simulink model "framework_sim"  (R2019b)
settings: Solver=FixedStepDiscrete  StartTime=T0  StopTime=Tf  FixedStep=Ts  EnableMultiTasking=on
model workspace (MAT data in the model file):
  aKalman = Simulink.Parameter
  aKalman.DataType = 'auto'
  aKalman.Dimensions = [0 0]
  slipEnabler = Simulink.Parameter
  slipEnabler.DataType = 'auto'
  slipEnabler.Dimensions = [0 0]
values from neighbouring files (symbols this model uses):
  enable_onlinePlots = 0    [main_framework.m]
  enable_zoom = 0    [main_framework.m]
  HLP_sampleTime = planner.replan_time    [main_framework.m]
  Kb = 10    [main_framework.m]
  Kd_vals = PID_Gain_Scheduling(:,4)    [main_framework.m]
  Ki_vals = PID_Gain_Scheduling(:,3)    [main_framework.m]
  Kp_vals = PID_Gain_Scheduling(:,2)    [main_framework.m]
  latContr_select = 4    [select_lateralController.m]
  mapObjects = scenario.scenario_data.mapObjects    [main_framework.m]
  N_vals = PID_Gain_Scheduling(:,5)    [main_framework.m]
  refRoute_fewPoints = referencePath_fewPoints.refRoute_fewPoints    [main_framework.m]    (also in refPath_poses_fewPoints.mat = [5 34.9682620653 63.3276365473 92.153562059 121.414282249 15; routePlanner.m = [x_cloth_refPath_fewPoints',y_cloth_refPath_fewPoints',theta)
  speed_vals_PID_sched = PID_Gain_Scheduling(:,1)    [main_framework.m]
  tau_D = vehicle_data.steering_system.tau_D    [dataAnalysis.m]    (also in main_framework.m)
  Ts = simulationPars.times.step_size    [main_framework.m]
  vehicle_data = getVehicleDataStruct()    [aeroModel.m]    (also in loadInitialConditions.m; longitSlipModel.m; main_framework.m; perfectAcker.m)
  X0 = loadInitialConditions    [main_framework.m]
undefined symbols (not defined in the file or in its folder): DiscIntNeverNeededParam, loadInitialPose
libraries: simulink_extras x16, drivingvehiclecontroller x2, simulink x1
(part 1 of 3)
settings Model: Creator=Edoardo  LastModifiedBy=Alvaro
settings DataIOCC: SaveFormat=Array  ReturnWorkspaceOutputs=off
settings OptimizationCC: DefaultParameterBehavior=Inlined  PassReuseOutputArgsAs=Individual arguments  MaxStackSize=64  EfficientTunableParamExpr=on
settings DebuggingCC: ReadBeforeWriteMsg=DisableAll  WriteAfterWriteMsg=DisableAll  WriteAfterReadMsg=DisableAll  MultiTaskDSMMsg=none  ParameterTunabilityLossMsg=error  PregeneratedLibrarySubsystemCodeDiagnostic=none  SFUnexpectedBacktrackingDiag=warning  SFNoUnconditionalDefaultTransitionDiag=warning  SFExecutionAtInitializationDiag=none  ArithmeticOperatorsInVariantConditions=warning
settings HardwareCC: ProdBitPerInt=16  ProdBitPerPointer=16  ProdBitPerSizeT=16  ProdBitPerPtrDiffT=16  ProdLargestAtomicFloat=None  ProdWordSize=16  ProdHWDeviceType=STMicroelectronics->ST10/Super10
settings ModelReferenceCC: UpdateModelReferenceTargets=IfOutOfDate  PropagateSignalLabelsOutOfModel=off
settings SFSimCC: SFSimEcho=off  SimUseLocalCustomCode=off  MATLABDynamicMemAlloc=off  CustomCodeUndefinedFunction=UseInterfaceOnly
settings RTWCC: SystemTargetFile=ert.tlc  TemplateMakefile=ert_default_tmf  GenerateReport=on  RetainRTWFile=on  RTWUseLocalCustomCode=off  Toolchain=GNU Tools for ARM Embedded Processors  BuildConfiguration=Faster Runs  IncludeHyperlinkInReport=on  LaunchReport=on  GenerateTraceInfo=on  GenerateTraceReport=on  GenerateTraceReportSl=on  GenerateTraceReportSf=on  GenerateTraceReportEml=on
settings CodeAppCC: ForceParamTrailComments=on  IgnoreCustomStorageClasses=off  OperatorAnnotations=on  SimulinkDataObjDesc=on  SFDataObjDesc=on  InsertBlockDesc=on
settings ERTTargetCC: CodeReplacementLibrary=ARM Cortex-M (Optimized)  SupportVariableSizeSignals=on  RootIOFormat=Structure reference  ERTCustomFileTemplate=example_file_process.tlc
settings ConfigComp: CovMetricSettings=dw  CovHtmlReporting=on  CovSaveCumulativeToWorkspaceVar=on  CovSaveSingleToWorkspaceVar=on  CovExternalEMLEnable=off

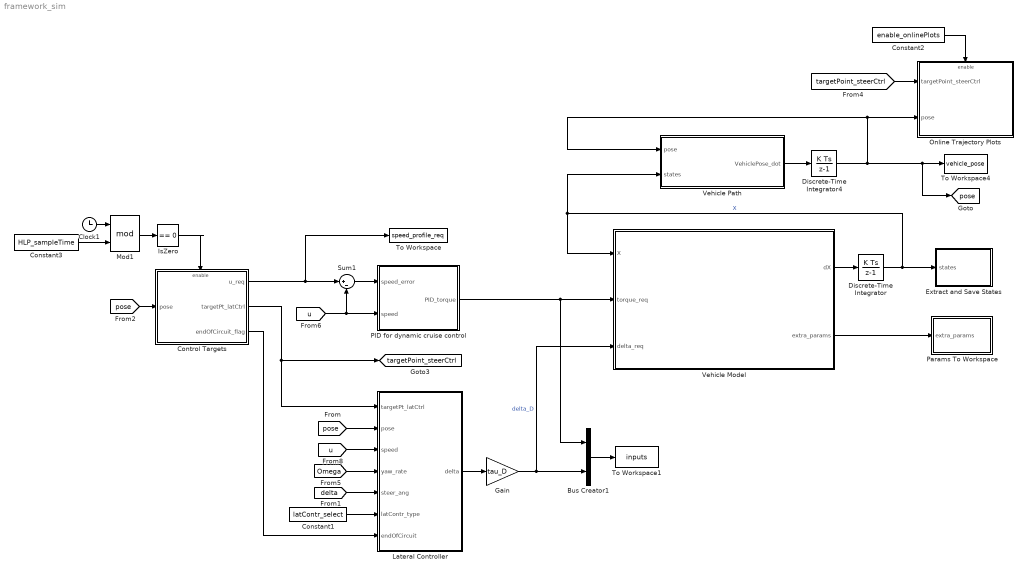
== system framework_sim ==
  Bus Creator1 : BusCreator  Inputs=2
  Clock1 : Clock
  Constant1 : Constant  Value=latContr_select
  Constant2 : Constant  Value=enable_onlinePlots
  Constant3 : Constant  Value=HLP_sampleTime
  Control Targets : Subsystem
  Discrete-Time Integrator : DiscreteIntegrator  gainval=1  InitialCondition=X0  SampleTime=-1  ICPrevOutput=DiscIntNeverNeededParam  ICPrevScaledInput=DiscIntNeverNeededParam
  Discrete-Time Integrator4 : DiscreteIntegrator  gainval=1  InitialCondition=loadInitialPose  SampleTime=-1  ICPrevOutput=DiscIntNeverNeededParam  ICPrevScaledInput=DiscIntNeverNeededParam
  Extract and Save States : Subsystem
  Gain : Gain  Gain=tau_D
  IsZero : simulink/Logic and Bit Operations/Compare To Zero  relop===  OutDataTypeStr=boolean
  Lateral Controller : Subsystem
  Mod1 : Math  Operator=mod  SaturateOnIntegerOverflow=on
  Online Trajectory Plots : Subsystem
      mask Display: image('/Users/mattiapiccinini/Documents/Google_Drive/PhD/Didattica/VDPC_EIT_2019_2020/Homework/Matlab_Maple/Homework_Autonomous_Drive_EIT/Scenario/example_path.png'); % Use "Edit Image" on toolstrip to change.
  PID for dynamic cruise control : Subsystem
  Params To Workspace : Subsystem
  Sum1 : Sum  Inputs=|+-
  To Workspace : ToWorkspace  VariableName=speed_profile_req  SaveFormat=Timeseries  SampleTime=-1
      settings: Save2DSignal=2-D array (concatenate along first dimension)
  To Workspace1 : ToWorkspace  VariableName=inputs  SaveFormat=Timeseries  SampleTime=-1
  To Workspace4 : ToWorkspace  VariableName=vehicle_pose  SampleTime=-1
      settings: Save2DSignal=2-D array (concatenate along first dimension)
  Vehicle Model : MATLAB Function  TreatAsAtomicUnit=on
  Vehicle Path : MATLAB Function  TreatAsAtomicUnit=on
  tag scope: pose=global, targetPoint_steerCtrl=global
  wires:
  [u] -> Sum1/2, PID for dynamic cruise control/2(speed)
  Vehicle Model/2(extra_params) -> Params To Workspace/1(extra_params)
  Discrete-Time Integrator/1 -> Extract and Save States/1(states), Vehicle Model/1(X), Vehicle Path/2(states)  "X"
  Vehicle Path/1(VehiclePose_dot) -> Discrete-Time Integrator4/1
  Discrete-Time Integrator4/1 -> [pose], To Workspace4/1, Online Trajectory Plots/2(pose), Vehicle Path/1(pose)
  Vehicle Model/1(dX) -> Discrete-Time Integrator/1
  Bus Creator1/1 -> To Workspace1/1
  PID for dynamic cruise control/1(PID_torque) -> Bus Creator1/1, Vehicle Model/2(torque_req)
  Sum1/1 -> PID for dynamic cruise control/1(speed_error)
  [targetPoint_steerCtrl] -> Online Trajectory Plots/1(targetPoint_steerCtrl)
  Gain/1 -> Vehicle Model/3(delta_req), Bus Creator1/2  "delta_D"
  Constant2/1 -> Online Trajectory Plots/Enable
  [pose] -> Lateral Controller/2(pose)
  [u] -> Lateral Controller/3(speed)
  Lateral Controller/1(delta) -> Gain/1
  Constant1/1 -> Lateral Controller/6(latContr_type)
  [Omega] -> Lateral Controller/4(yaw_rate)
  [delta] -> Lateral Controller/5(steer_ang)
  Control Targets/2(targetPt_latCtrl) -> Lateral Controller/1(targetPt_latCtrl), [targetPoint_steerCtrl]
  Control Targets/1(u_req) -> To Workspace/1, Sum1/1
  [pose] -> Control Targets/1(pose)
  Clock1/1 -> Mod1/1
  Constant3/1 -> Mod1/2
  Mod1/1 -> IsZero/1
  IsZero/1 -> Control Targets/Enable
  Control Targets/3(endOfCircuit_flag) -> Lateral Controller/7(endOfCircuit)

== system framework_sim/Control Targets ==
  pose : Inport
  Enable : EnablePort
  MATLAB System : MATLABSystem  System=setControlTargets  lateralController_type=latContr_select  purePursuit_lookAhead=purePursuitParams.lookAhead  clothoidBased_lookAhead=clothoidBasedParams.lookAhead  refRoute_points=refRoute_fewPoints  Lf=vehicle_data.vehicle.Lf  x_parkLot=mapObjects(1,1)  y_lowBound_parkLot=mapObjects(2,2)  y_uppBound_parkLot=mapObjects(1,2)  SimulateUsing=Interpreted execution
      mask Type: setControlTargets
      mask Display:
      | disp('setControlTargets');
      | port_label('input',1,'vehPose');
      | port_label('output',1,'targetPoint_latControl');
      | port_label('output',2,'speed_req');
      | port_label('output',3,'endOfCircuit');
  u_req : Outport  VectorParamsAs1DForOutWhenUnconnected=off
  targetPt_latCtrl : Outport  Port=2  VectorParamsAs1DForOutWhenUnconnected=off
  endOfCircuit_flag : Outport  Port=3  VectorParamsAs1DForOutWhenUnconnected=off
  wires:
  pose/1 -> MATLAB System/1
  MATLAB System/2 -> u_req/1
  MATLAB System/1 -> targetPt_latCtrl/1
  MATLAB System/3 -> endOfCircuit_flag/1

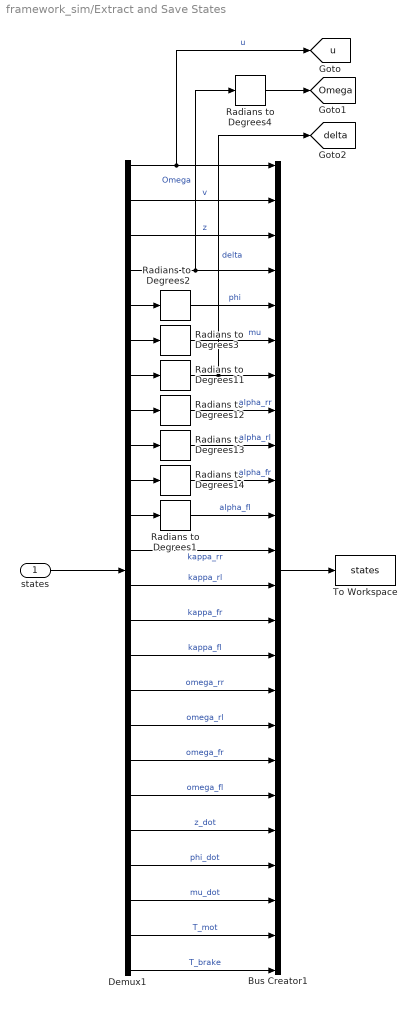
== system framework_sim/Extract and Save States ==
  states : Inport
  Bus Creator1 : BusCreator  Inputs=24
  Demux1 : Demux  Outputs=24
  Radians to Degrees{1..4,11..14} (8 alike) : simulink_extras/Transformations/Radians to Degrees
  To Workspace : ToWorkspace  VariableName=states  SaveFormat=Timeseries  SampleTime=-1
  tag scope: Omega=global, delta=global, u=global
  wires:
  Demux1/24 -> Bus Creator1/24  "T_brake"
  Demux1/13 -> Bus Creator1/13  "kappa_rl"
  Radians to Degrees12/1 -> Bus Creator1/8  "alpha_rr"
  Demux1/6 -> Radians to Degrees3/1
  Demux1/23 -> Bus Creator1/23  "T_mot"
  Demux1/19 -> Bus Creator1/19  "omega_fl"
  Demux1/8 -> Radians to Degrees12/1
  states/1 -> Demux1/1
  Demux1/14 -> Bus Creator1/14  "kappa_fr"
  Demux1/9 -> Radians to Degrees13/1
  Radians to Degrees11/1 -> Bus Creator1/7, [delta]  "delta"
  Demux1/15 -> Bus Creator1/15  "kappa_fl"
  Demux1/3 -> Bus Creator1/3  "z"
  Demux1/22 -> Bus Creator1/22  "mu_dot"
  Demux1/4 -> Bus Creator1/4, Radians to Degrees4/1  "Omega"
  Radians to Degrees3/1 -> Bus Creator1/6  "mu"
  Radians to Degrees1/1 -> Bus Creator1/11  "alpha_fl"
  Radians to Degrees2/1 -> Bus Creator1/5  "phi"
  Radians to Degrees13/1 -> Bus Creator1/9  "alpha_rl"
  Demux1/5 -> Radians to Degrees2/1
  Demux1/21 -> Bus Creator1/21  "phi_dot"
  Demux1/7 -> Radians to Degrees11/1
  Demux1/12 -> Bus Creator1/12  "kappa_rr"
  Demux1/17 -> Bus Creator1/17  "omega_rl"
  Demux1/2 -> Bus Creator1/2  "v"
  Demux1/20 -> Bus Creator1/20  "z_dot"
  Demux1/10 -> Radians to Degrees14/1
  Demux1/11 -> Radians to Degrees1/1
  Radians to Degrees14/1 -> Bus Creator1/10  "alpha_fr"
  Demux1/18 -> Bus Creator1/18  "omega_fr"
  Demux1/1 -> [u], Bus Creator1/1  "u"
  Demux1/16 -> Bus Creator1/16  "omega_rr"
  Bus Creator1/1 -> To Workspace/1
  Radians to Degrees4/1 -> [Omega]

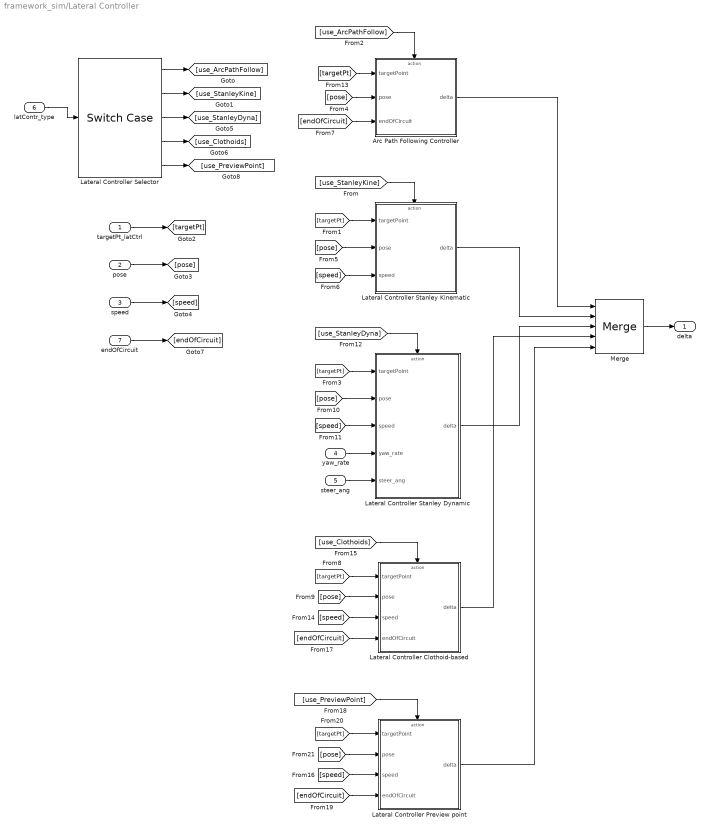
== system framework_sim/Lateral Controller ==
  targetPt_latCtrl : Inport
  pose : Inport  Port=2
  speed : Inport  Port=3
  yaw_rate : Inport  Port=4
  steer_ang : Inport  Port=5
  latContr_type : Inport  Port=6
  endOfCircuit : Inport  Port=7
  Arc Path Following Controller : Subsystem  TreatAsAtomicUnit=on
  Lateral Controller Clothoid-based : Subsystem  TreatAsAtomicUnit=on
  Lateral Controller Preview point : Subsystem  TreatAsAtomicUnit=on
  Lateral Controller Selector : SwitchCase  CaseConditions={1,2,3,4,5}  ShowDefaultCase=off
  Lateral Controller Stanley Dynamic : Subsystem  TreatAsAtomicUnit=on
  Lateral Controller Stanley Kinematic : Subsystem  TreatAsAtomicUnit=on
  Merge : Merge  Inputs=5
  delta : Outport  VectorParamsAs1DForOutWhenUnconnected=off
  wires:
  Arc Path Following Controller/1(delta) -> Merge/1
  latContr_type/1 -> Lateral Controller Selector/1
  Lateral Controller Stanley Kinematic/1(delta) -> Merge/2
  Merge/1 -> delta/1
  Lateral Controller Selector/1 -> [use_ArcPathFollow]
  [use_ArcPathFollow] -> Arc Path Following Controller/Action
  Lateral Controller Selector/2 -> [use_StanleyKine]
  [use_StanleyKine] -> Lateral Controller Stanley Kinematic/Action
  targetPt_latCtrl/1 -> [targetPt]
  [targetPt] -> Arc Path Following Controller/1(targetPoint)
  [targetPt] -> Lateral Controller Stanley Kinematic/1(targetPoint)
  pose/1 -> [pose]
  [pose] -> Arc Path Following Controller/2(pose)
  [pose] -> Lateral Controller Stanley Kinematic/2(pose)
  speed/1 -> [speed]
  [speed] -> Lateral Controller Stanley Kinematic/3(speed)
  Lateral Controller Selector/3 -> [use_StanleyDyna]
  [pose] -> Lateral Controller Stanley Dynamic/2(pose)
  [targetPt] -> Lateral Controller Stanley Dynamic/1(targetPoint)
  [speed] -> Lateral Controller Stanley Dynamic/3(speed)
  [use_StanleyDyna] -> Lateral Controller Stanley Dynamic/Action
  Lateral Controller Stanley Dynamic/1(delta) -> Merge/3
  yaw_rate/1 -> Lateral Controller Stanley Dynamic/4(yaw_rate)
  steer_ang/1 -> Lateral Controller Stanley Dynamic/5(steer_ang)
  [use_Clothoids] -> Lateral Controller Clothoid-based/Action
  [pose] -> Lateral Controller Clothoid-based/2(pose)
  [targetPt] -> Lateral Controller Clothoid-based/1(targetPoint)
  [speed] -> Lateral Controller Clothoid-based/3(speed)
  Lateral Controller Clothoid-based/1(delta) -> Merge/4
  Lateral Controller Selector/4 -> [use_Clothoids]
  [endOfCircuit] -> Arc Path Following Controller/3(endOfCircuit)
  [endOfCircuit] -> Lateral Controller Clothoid-based/4(endOfCircuit)
  endOfCircuit/1 -> [endOfCircuit]
  Lateral Controller Selector/5 -> [use_PreviewPoint]
  [pose] -> Lateral Controller Preview point/2(pose)
  [endOfCircuit] -> Lateral Controller Preview point/4(endOfCircuit)
  [use_PreviewPoint] -> Lateral Controller Preview point/Action
  [speed] -> Lateral Controller Preview point/3(speed)
  [targetPt] -> Lateral Controller Preview point/1(targetPoint)
  Lateral Controller Preview point/1(delta) -> Merge/5

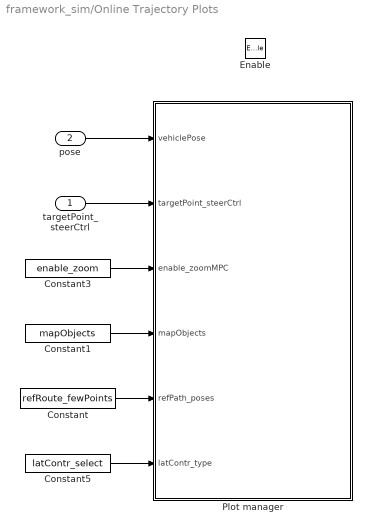
== system framework_sim/Online Trajectory Plots ==
  targetPoint_steerCtrl : Inport
  pose : Inport  Port=2
  Enable : EnablePort
  Constant : Constant  Value=refRoute_fewPoints
  Constant1 : Constant  Value=mapObjects
  Constant3 : Constant  Value=enable_zoom
  Constant5 : Constant  Value=latContr_select
  Plot manager : MATLAB Function  TreatAsAtomicUnit=on
  wires:
  targetPoint_steerCtrl/1 -> Plot manager/2(targetPoint_steerCtrl)
  Constant/1 -> Plot manager/5(refPath_poses)
  Constant3/1 -> Plot manager/3(enable_zoomMPC)
  pose/1 -> Plot manager/1(vehiclePose)
  Constant1/1 -> Plot manager/4(mapObjects)
  Constant5/1 -> Plot manager/6(latContr_type)

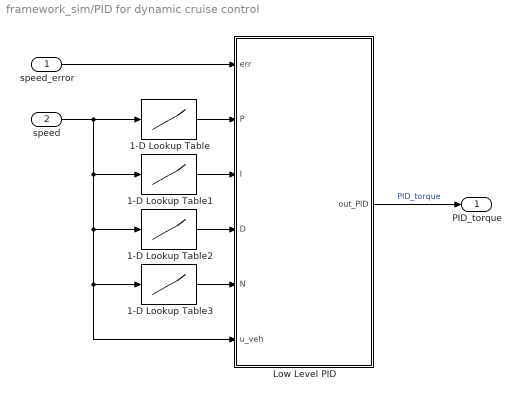
== system framework_sim/PID for dynamic cruise control ==
  speed_error : Inport
  speed : Inport  Port=2
  1-D Lookup Table : Lookup_n-D  NumberOfTableDimensions=1  BreakpointsForDimension1=speed_vals_PID_sched  BeginIndexSearchUsingPreviousIndexResult=on  Table=Kp_vals  ExtrapMethod=Clip  UseLastTableValue=on  InternalRulePriority=Speed  RndMeth=Simplest  InputSameDT=on
  1-D Lookup Table1 : Lookup_n-D  NumberOfTableDimensions=1  BreakpointsForDimension1=speed_vals_PID_sched  BeginIndexSearchUsingPreviousIndexResult=on  Table=Ki_vals  ExtrapMethod=Clip  UseLastTableValue=on  InternalRulePriority=Speed  RndMeth=Simplest  InputSameDT=on
  1-D Lookup Table2 : Lookup_n-D  NumberOfTableDimensions=1  BreakpointsForDimension1=speed_vals_PID_sched  BeginIndexSearchUsingPreviousIndexResult=on  Table=Kd_vals  ExtrapMethod=Clip  UseLastTableValue=on  InternalRulePriority=Speed  RndMeth=Simplest  InputSameDT=on
  1-D Lookup Table3 : Lookup_n-D  NumberOfTableDimensions=1  BreakpointsForDimension1=speed_vals_PID_sched  BeginIndexSearchUsingPreviousIndexResult=on  Table=N_vals  ExtrapMethod=Clip  UseLastTableValue=on  InternalRulePriority=Speed  RndMeth=Simplest  InputSameDT=on
  Low Level PID : Subsystem
  PID_torque : Outport  VectorParamsAs1DForOutWhenUnconnected=off
  wires:
  1-D Lookup Table1/1 -> Low Level PID/3(I)
  speed_error/1 -> Low Level PID/1(err)
  speed/1 -> Low Level PID/6(u_veh), 1-D Lookup Table3/1, 1-D Lookup Table2/1, 1-D Lookup Table1/1, 1-D Lookup Table/1
  1-D Lookup Table3/1 -> Low Level PID/5(N)
  Low Level PID/1(out_PID) -> PID_torque/1  "PID_torque"
  1-D Lookup Table/1 -> Low Level PID/2(P)
  1-D Lookup Table2/1 -> Low Level PID/4(D)

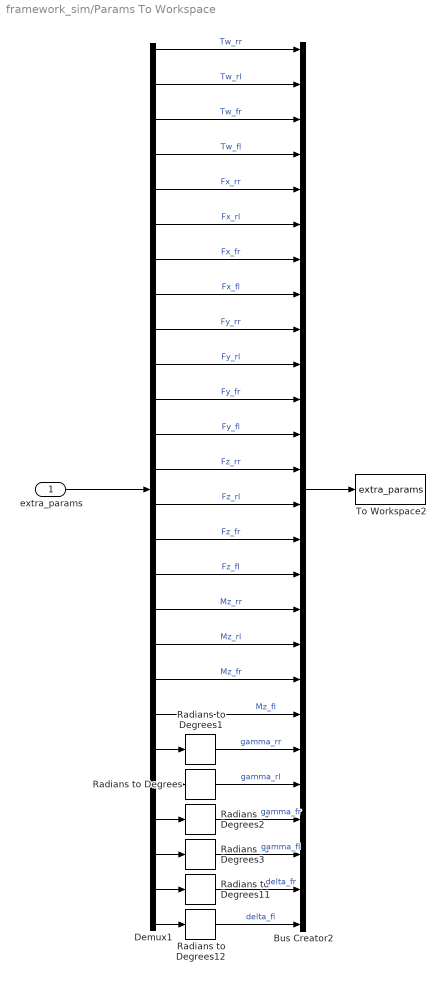
== system framework_sim/Params To Workspace ==
  extra_params : Inport
  Bus Creator2 : BusCreator  Inputs=26
  Demux1 : Demux  Outputs=26
  Radians to Degrees{,1..3,11..12} (6 alike) : simulink_extras/Transformations/Radians to Degrees
  To Workspace2 : ToWorkspace  VariableName=extra_params  SaveFormat=Timeseries  SampleTime=-1
  wires:
  Demux1/16 -> Bus Creator2/16  "Fz_fl"
  Demux1/21 -> Radians to Degrees1/1
  Demux1/3 -> Bus Creator2/3  "Tw_fr"
  Demux1/22 -> Radians to Degrees/1
  Demux1/23 -> Radians to Degrees2/1
  Radians to Degrees3/1 -> Bus Creator2/24  "gamma_fl"
  Demux1/20 -> Bus Creator2/20  "Mz_fl"
  Radians to Degrees1/1 -> Bus Creator2/21  "gamma_rr"
  Radians to Degrees11/1 -> Bus Creator2/25  "delta_fr"
  Demux1/18 -> Bus Creator2/18  "Mz_rl"
  Demux1/13 -> Bus Creator2/13  "Fz_rr"
  Demux1/4 -> Bus Creator2/4  "Tw_fl"
  Demux1/6 -> Bus Creator2/6  "Fx_rl"
  Demux1/8 -> Bus Creator2/8  "Fx_fl"
  Demux1/17 -> Bus Creator2/17  "Mz_rr"
  Demux1/7 -> Bus Creator2/7  "Fx_fr"
  Demux1/5 -> Bus Creator2/5  "Fx_rr"
  Demux1/9 -> Bus Creator2/9  "Fy_rr"
  Demux1/24 -> Radians to Degrees3/1
  Demux1/26 -> Radians to Degrees12/1
  Demux1/11 -> Bus Creator2/11  "Fy_fr"
  Demux1/19 -> Bus Creator2/19  "Mz_fr"
  Demux1/10 -> Bus Creator2/10  "Fy_rl"
  Radians to Degrees12/1 -> Bus Creator2/26  "delta_fl"
  Radians to Degrees2/1 -> Bus Creator2/23  "gamma_fr"
  extra_params/1 -> Demux1/1
  Demux1/12 -> Bus Creator2/12  "Fy_fl"
  Bus Creator2/1 -> To Workspace2/1
  Demux1/15 -> Bus Creator2/15  "Fz_fr"
  Demux1/25 -> Radians to Degrees11/1
  Demux1/1 -> Bus Creator2/1  "Tw_rr"
  Demux1/2 -> Bus Creator2/2  "Tw_rl"
  Demux1/14 -> Bus Creator2/14  "Fz_rl"
  Radians to Degrees/1 -> Bus Creator2/22  "gamma_rl"

== system framework_sim/Lateral Controller/Arc Path Following Controller ==
  targetPoint : Inport
  pose : Inport  Port=2
  endOfCircuit : Inport  Port=3
  Action Port : ActionPort  ActionPortLabel=case [ 1 ]:
  Arc Path Following Controller : MATLAB Function  TreatAsAtomicUnit=on
  delta : Outport  VectorParamsAs1DForOutWhenUnconnected=off
  wires:
  Arc Path Following Controller/1(delta) -> delta/1
  targetPoint/1 -> Arc Path Following Controller/1(target_Point)
  pose/1 -> Arc Path Following Controller/2(pose)
  endOfCircuit/1 -> Arc Path Following Controller/3(endOfCircuit)

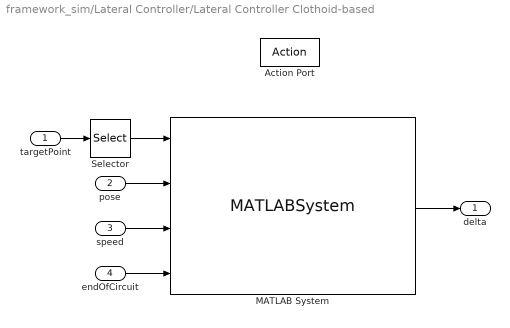
== system framework_sim/Lateral Controller/Lateral Controller Clothoid-based ==
  targetPoint : Inport
  pose : Inport  Port=2
  speed : Inport  Port=3
  endOfCircuit : Inport  Port=4
  Action Port : ActionPort  ActionPortLabel=case [ 4 ]:
  MATLAB System : MATLABSystem  System=clothoidBased_lateralController  lookAhead=clothoidBasedParams.lookAhead  Kus=clothoidBasedParams.Kus  L=vehicle_data.vehicle.L  SimulateUsing=Interpreted execution
      mask Type: clothoidBased_lateralController
      mask Display:
      | disp('clothoidBased_lateralController');
      | port_label('input',1,'targetPoint');
      | port_label('input',2,'vehPose');
      | port_label('input',3,'vehSpeed');
      | port_label('input',4,'endOfCircuit');
      | port_label('output',1,'delta_req');
  Selector : Selector  InputPortWidth=4  IndexOptions=Index vector (dialog)  Indices=[1 2 3]  OutputSizes=1
  delta : Outport  VectorParamsAs1DForOutWhenUnconnected=off
  wires:
  speed/1 -> MATLAB System/3
  MATLAB System/1 -> delta/1
  pose/1 -> MATLAB System/2
  targetPoint/1 -> Selector/1
  Selector/1 -> MATLAB System/1
  endOfCircuit/1 -> MATLAB System/4

== system framework_sim/Lateral Controller/Lateral Controller Preview point ==
  targetPoint : Inport
  pose : Inport  Port=2
  speed : Inport  Port=3
  endOfCircuit : Inport  Port=4
  Action Port : ActionPort  ActionPortLabel=case [ 4 ]:
  MATLAB System : MATLABSystem  System=clothoidBased_lateralController  lookAhead=clothoidBasedParams.lookAhead  Kus=clothoidBasedParams.Kus  L=vehicle_data.vehicle.L  SimulateUsing=Interpreted execution
      mask Type: clothoidBased_lateralController
      mask Display:
      | disp('clothoidBased_lateralController');
      | port_label('input',1,'targetPoint');
      | port_label('input',2,'vehPose');
      | port_label('input',3,'vehSpeed');
      | port_label('input',4,'endOfCircuit');
      | port_label('output',1,'delta_req');
  Selector : Selector  InputPortWidth=4  IndexOptions=Index vector (dialog)  Indices=[1 2 3]  OutputSizes=1
  delta : Outport  VectorParamsAs1DForOutWhenUnconnected=off
  wires:
  speed/1 -> MATLAB System/3
  MATLAB System/1 -> delta/1
  pose/1 -> MATLAB System/2
  targetPoint/1 -> Selector/1
  Selector/1 -> MATLAB System/1
  endOfCircuit/1 -> MATLAB System/4

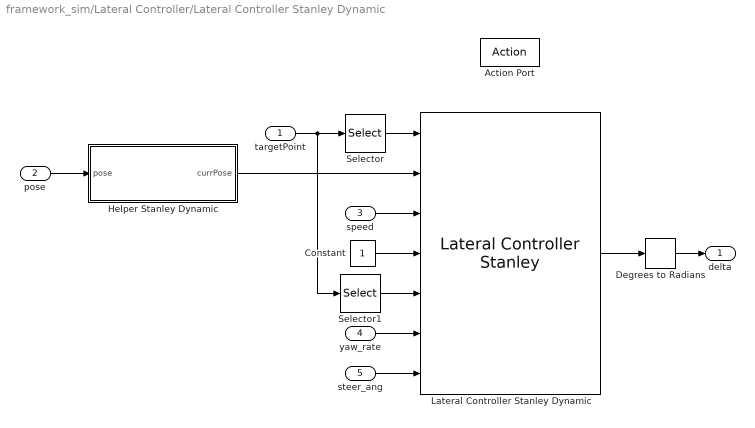
== system framework_sim/Lateral Controller/Lateral Controller Stanley Dynamic ==
  targetPoint : Inport
  pose : Inport  Port=2
  speed : Inport  Port=3
  yaw_rate : Inport  Port=4
  steer_ang : Inport  Port=5
  Action Port : ActionPort  ActionPortLabel=case [ 3 ]:
  Constant : Constant
  Degrees to Radians : simulink_extras/Transformations/Degrees to Radians
  Helper Stanley Dynamic : MATLAB Function  TreatAsAtomicUnit=on
  Lateral Controller Stanley Dynamic : drivingvehiclecontroller/Lateral Controller Stanley  ModelType=Dynamic bicycle model  PositionGainF=stanleyParams.positGainFW  PositionGainR=stanleyParams.positGainREV  YawRateGain=stanleyParams.yawRateGain  DelayGain=stanleyParams.steerGain  VehicleMass=vehicle_data.vehicle.m  Lf=vehicle_data.vehicle.Lf  Lr=vehicle_data.vehicle.Lr  TireStiffness=stanleyParams.cornerStiff  Wheelbase=vehicleDims.Wheelbase  MaxSteeringAngle=stanleyParams.maxSteerAngle
      settings: SourceProductName=Automated Driving Toolbox  SourceProductBaseCode=DR
  Selector : Selector  InputPortWidth=4  IndexOptions=Index vector (dialog)  Indices=[1 2 3]  OutputSizes=1
  Selector1 : Selector  InputPortWidth=4  IndexOptions=Index vector (dialog)  Indices=[4]  OutputSizes=1
  delta : Outport  VectorParamsAs1DForOutWhenUnconnected=off
  wires:
  Lateral Controller Stanley Dynamic/1 -> Degrees to Radians/1
  pose/1 -> Helper Stanley Dynamic/1(pose)
  speed/1 -> Lateral Controller Stanley Dynamic/3
  Constant/1 -> Lateral Controller Stanley Dynamic/4
  Degrees to Radians/1 -> delta/1
  Helper Stanley Dynamic/1(currPose) -> Lateral Controller Stanley Dynamic/2
  yaw_rate/1 -> Lateral Controller Stanley Dynamic/6
  steer_ang/1 -> Lateral Controller Stanley Dynamic/7
  targetPoint/1 -> Selector/1, Selector1/1
  Selector/1 -> Lateral Controller Stanley Dynamic/1
  Selector1/1 -> Lateral Controller Stanley Dynamic/5

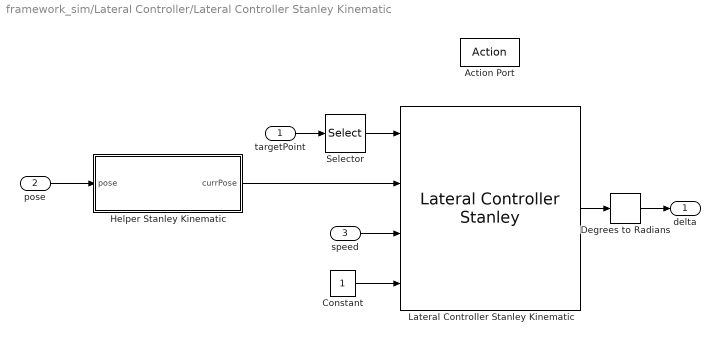
== system framework_sim/Lateral Controller/Lateral Controller Stanley Kinematic ==
  targetPoint : Inport
  pose : Inport  Port=2
  speed : Inport  Port=3
  Action Port : ActionPort  ActionPortLabel=case [ 2 ]:
  Constant : Constant
  Degrees to Radians : simulink_extras/Transformations/Degrees to Radians
  Helper Stanley Kinematic : MATLAB Function  TreatAsAtomicUnit=on
  Lateral Controller Stanley Kinematic : drivingvehiclecontroller/Lateral Controller Stanley  ModelType=Kinematic bicycle model  PositionGainF=stanleyParams.positGainFW  PositionGainR=stanleyParams.positGainREV  YawRateGain=0.2  DelayGain=0.2  VehicleMass=1575  Lf=1.2  Lr=1.6  TireStiffness=19000  Wheelbase=vehicleDims.Wheelbase  MaxSteeringAngle=stanleyParams.maxSteerAngle
      settings: SourceProductName=Automated Driving Toolbox  SourceProductBaseCode=DR
  Selector : Selector  InputPortWidth=4  IndexOptions=Index vector (dialog)  Indices=[1 2 3]  OutputSizes=1
  delta : Outport  VectorParamsAs1DForOutWhenUnconnected=off
  wires:
  Lateral Controller Stanley Kinematic/1 -> Degrees to Radians/1
  pose/1 -> Helper Stanley Kinematic/1(pose)
  speed/1 -> Lateral Controller Stanley Kinematic/3
  Constant/1 -> Lateral Controller Stanley Kinematic/4
  Degrees to Radians/1 -> delta/1
  Helper Stanley Kinematic/1(currPose) -> Lateral Controller Stanley Kinematic/2
  targetPoint/1 -> Selector/1
  Selector/1 -> Lateral Controller Stanley Kinematic/1

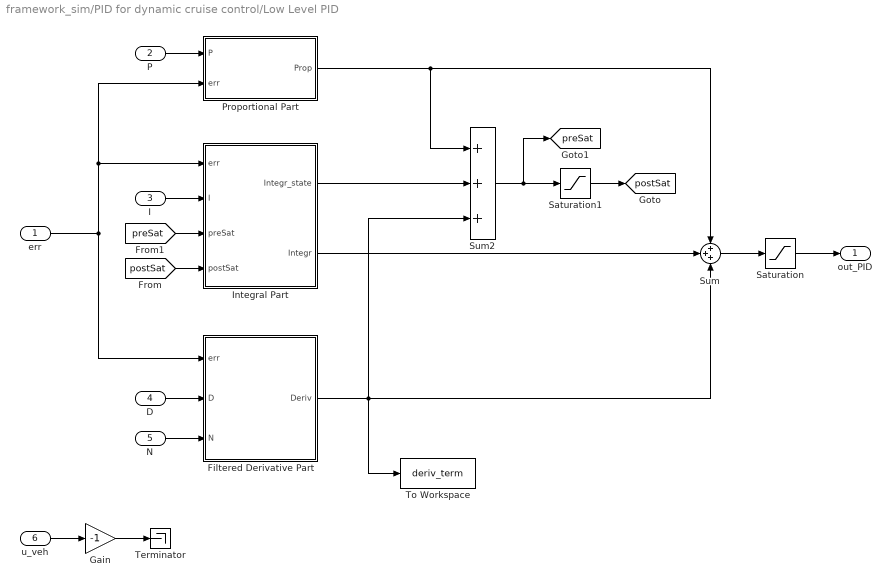
== system framework_sim/PID for dynamic cruise control/Low Level PID ==
  err : Inport
  P : Inport  Port=2
  I : Inport  Port=3
  D : Inport  Port=4
  N : Inport  Port=5
  u_veh : Inport  Port=6
  Filtered Derivative Part : Subsystem
  Gain : Gain  Gain=-1
  Integral Part : Subsystem
  Proportional Part : Subsystem
  Saturation : Saturate  UpperLimit=vehicle_data.motor.maxTorque  LowerLimit=-vehicle_data.braking.totBrakeTorque*vehicle_data.braking.brakeRatio  LinearizeAsGain=off
  Saturation1 : Saturate  UpperLimit=vehicle_data.motor.maxTorque  LowerLimit=-vehicle_data.braking.totBrakeTorque*vehicle_data.braking.brakeRatio  LinearizeAsGain=off
  Sum : Sum  Inputs=+++
  Sum2 : Sum  Inputs=+++
  Terminator : Terminator
  To Workspace : ToWorkspace  VariableName=deriv_term  SaveFormat=Timeseries  SampleTime=Ts
  out_PID : Outport  VectorParamsAs1DForOutWhenUnconnected=off
  tag scope: postSat=global, preSat=global
  wires:
  Sum2/1 -> [preSat], Saturation1/1
  Sum/1 -> Saturation/1
  Saturation/1 -> out_PID/1
  err/1 -> Filtered Derivative Part/1(err), Proportional Part/2(err), Integral Part/1(err)
  Saturation1/1 -> [postSat]
  I/1 -> Integral Part/2(I)
  Integral Part/1(Integr_state) -> Sum2/2
  Integral Part/2(Integr) -> Sum/2
  Proportional Part/1(Prop) -> Sum2/1, Sum/1
  P/1 -> Proportional Part/1(P)
  [preSat] -> Integral Part/3(preSat)
  [postSat] -> Integral Part/4(postSat)
  Filtered Derivative Part/1(Deriv) -> To Workspace/1, Sum/3, Sum2/3
  D/1 -> Filtered Derivative Part/2(D)
  N/1 -> Filtered Derivative Part/3(N)
  u_veh/1 -> Gain/1
  Gain/1 -> Terminator/1

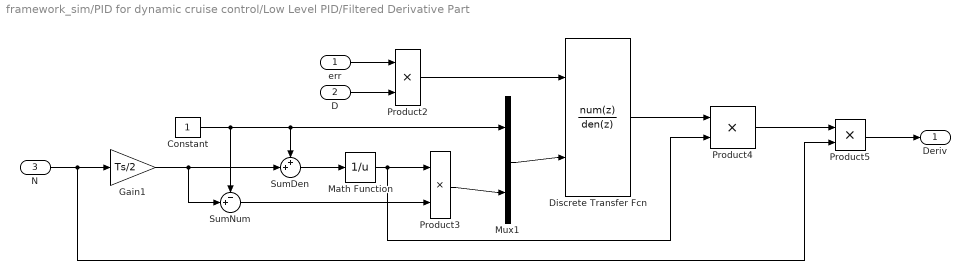
== system framework_sim/PID for dynamic cruise control/Low Level PID/Filtered Derivative Part ==
  err : Inport
  D : Inport  Port=2
  N : Inport  Port=3
  Constant : Constant
  Discrete Transfer Fcn : DiscreteTransferFcn  Numerator=[1 -1]  DenominatorSource=Input port  SampleTime=Ts  a0EqualsOne=on
      settings: InputPortMap=u0,p3
  Gain1 : Gain  Gain=Ts/2
  Math Function : Math  Operator=reciprocal  SaturateOnIntegerOverflow=on
  Mux1 : Mux  Inputs=2
  Product{2..5} (4 alike) : Product
  SumDen : Sum  Inputs=++|
  SumNum : Sum  Inputs=-+|
  Deriv : Outport  VectorParamsAs1DForOutWhenUnconnected=off
  wires:
  N/1 -> Gain1/1, Product5/2
  Product4/1 -> Product5/1
  SumDen/1 -> Math Function/1
  Math Function/1 -> Product4/2, Product3/1
  SumNum/1 -> Product3/2
  Product2/1 -> Discrete Transfer Fcn/1
  Discrete Transfer Fcn/1 -> Product4/1
  Constant/1 -> SumDen/1, Mux1/1, SumNum/1
  Product3/1 -> Mux1/2
  Mux1/1 -> Discrete Transfer Fcn/2
  Gain1/1 -> SumNum/2, SumDen/2
  err/1 -> Product2/1
  D/1 -> Product2/2
  Product5/1 -> Deriv/1

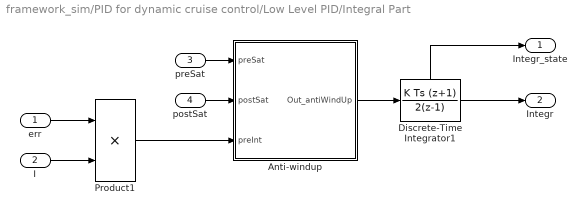
== system framework_sim/PID for dynamic cruise control/Low Level PID/Integral Part ==
  err : Inport
  I : Inport  Port=2
  preSat : Inport  Port=3
  postSat : Inport  Port=4
  Anti-windup : Subsystem
  Discrete-Time Integrator1 : DiscreteIntegrator  IntegratorMethod=Integration: Trapezoidal  SampleTime=Ts  ShowStatePort=on  ICPrevOutput=DiscIntNeverNeededParam  ICPrevScaledInput=DiscIntNeverNeededParam
  Product1 : Product
  Integr_state : Outport  VectorParamsAs1DForOutWhenUnconnected=off
  Integr : Outport  Port=2  VectorParamsAs1DForOutWhenUnconnected=off
  wires:
  Discrete-Time Integrator1/State -> Integr_state/1
  preSat/1 -> Anti-windup/1(preSat)
  Product1/1 -> Anti-windup/3(preInt)
  postSat/1 -> Anti-windup/2(postSat)
  I/1 -> Product1/2
  Anti-windup/1(Out_antiWindUp) -> Discrete-Time Integrator1/1
  Discrete-Time Integrator1/1 -> Integr/1
  err/1 -> Product1/1

== system framework_sim/PID for dynamic cruise control/Low Level PID/Proportional Part ==
  P : Inport
  err : Inport  Port=2
  Product : Product
  Prop : Outport  VectorParamsAs1DForOutWhenUnconnected=off
  wires:
  P/1 -> Product/2
  Product/1 -> Prop/1
  err/1 -> Product/1

== system framework_sim/PID for dynamic cruise control/Low Level PID/Integral Part/Anti-windup ==
  preSat : Inport
  postSat : Inport  Port=2
  preInt : Inport  Port=3
  Gain : Gain  Gain=Kb
  Sum : Sum  Inputs=|-+
  Sum1 : Sum  Inputs=|++
  Out_antiWindUp : Outport  VectorParamsAs1DForOutWhenUnconnected=off
  wires:
  preSat/1 -> Sum/1
  preInt/1 -> Sum1/2
  Gain/1 -> Sum1/1
  Sum1/1 -> Out_antiWindUp/1
  Sum/1 -> Gain/1
  postSat/1 -> Sum/2

== matlab function framework_sim/Lateral Controller/Lateral Controller Stanley Dynamic/Helper Stanley Dynamic ==
  data: pose input; currPose output
function currPose = helperStanleyDyn(pose)

    currPose = [pose(1), pose(2), rad2deg(pose(3))];

end

== matlab function framework_sim/Lateral Controller/Lateral Controller Stanley Kinematic/Helper Stanley Kinematic ==
  data: pose input; currPose output
function currPose = helperStanleyKine(pose)

    currPose = [pose(1), pose(2), rad2deg(pose(3))];

end

== matlab function framework_sim/Vehicle Path ==
  data: pose input; states input; VehiclePose_dot output
function VehiclePose_dot = VehiclePath(pose,states)

    u     = states(1);  % [m/s] longitudinal speed
    v     = states(2);  % [m/s] lateral speed
    Omega = states(4);  % [rad/s] yaw rate
    
    psi = pose(3);      % [rad] attitude
    
    x_dot   = u*cos(psi) - v*sin(psi);
    y_dot   = v*cos(psi) + u*sin(psi);
    psi_dot = Omega;

    VehiclePose_dot    = zeros(3,1);
    VehiclePose_dot(1) = x_dot;
    VehiclePose_dot(2) = y_dot;
    VehiclePose_dot(3) = psi_dot;

end

== matlab function framework_sim/Online Trajectory Plots/Plot manager ==
  data: vehiclePose input; targetPoint_steerCtrl input; enable_zoomMPC input; mapObjects input; refPath_poses input; latContr_type input
function real_time_plot(vehiclePose,targetPoint_steerCtrl,enable_zoomMPC,mapObjects,refPath_poses,latContr_type)
    
    coder.extrinsic('patch');
    
    %% Extract vehicle pose
    xCoMCar = vehiclePose(1);
    yCoMCar = vehiclePose(2);
    vehicleAttitude = vehiclePose(3);
    
    %% Load vehicle data
    vehicle_data = getVehicleDataStruct();
    Lf = vehicle_data.vehicle.Lf;        
    Lr = vehicle_data.vehicle.Lr;                 
    Wf = vehicle_data.vehicle.Wf;     
    Wr = vehicle_data.vehicle.Wr;
    
    %% Delete the plots for the previous iteration
    cla;
    
    %% Sketch the vehicle and its position, for this MPC iteration
    % Rotation matrix from vehicle (mobile) frame to the absolute frame
    RotMat = [cos(vehicleAttitude), -sin(vehicleAttitude); ...
              sin(vehicleAttitude), cos(vehicleAttitude)];
    
    pos_vehRR = RotMat*[-Lr -Wr/2]';
    pos_vehRL = RotMat*[-Lr +Wr/2]';
    pos_vehFR = RotMat*[+Lf -Wf/2]';
    pos_vehFL = RotMat*[+Lf +Wf/2]';
    pos_veh   = [pos_vehRR pos_vehRL pos_vehFL pos_vehFR];
    
    % Current vehicle pose
    patch(xCoMCar + pos_veh(1,:),yCoMCar + pos_veh(2,:),'yellow');
    
    % Optimal route computed with route planner
    X_route = refPath_poses(:,1);
    Y_route = refPath_poses(:,2);
    plot(X_route,Y_route,'go','MarkerSize',2)
    
    % Objects of the road scenario (walls, fixed obstacles etc)
    for ii=1:size(mapObjects,1)
        rectangle('Position',mapObjects(ii,:),'FaceColor',color('purple'),'EdgeColor',color('purple'),'LineWidth',2)
    end
    
    % Target point used by some low-level lateral controllers
    if (latContr_type==1 || latContr_type==4)  
        plot(targetPoint_steerCtrl(1),targetPoint_steerCtrl(2),'r*','MarkerSize',6)
    end
    
    % Zoom on the vehicle if required
    if (enable_zoomMPC)
        xlim([xCoMCar-40 xCoMCar+40])
        ylim([yCoMCar-40 yCoMCar+40])
    end
    
end
